simulink model "Octocopter2DLin"  (R2017b)
settings: Solver=VariableStepAuto  StartTime=0.0  StopTime=20  RelTol=1e-3
undefined symbols (not defined in the file): A, ACmp, B1, B2, BCmp, C2, CCmp, D21, DCmp, xInit
settings Model: Creator=jeremie  LastModifiedBy=jeremie

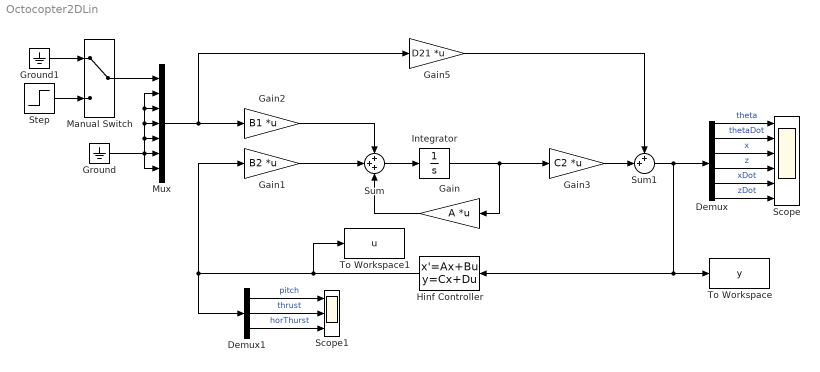
== system Octocopter2DLin ==
  Demux : Demux  Outputs=6
  Demux1 : Demux  Outputs=3
  Gain : Gain  Gain=A  Multiplication=Matrix(K*u)
  Gain1 : Gain  Gain=B2  Multiplication=Matrix(K*u)
  Gain2 : Gain  Gain=B1  Multiplication=Matrix(K*u)
  Gain3 : Gain  Gain=C2  Multiplication=Matrix(K*u)
  Gain5 : Gain  Gain=D21  Multiplication=Matrix(K*u)
  Ground : Ground
  Ground1 : Ground
  Hinf Controller : StateSpace  A=ACmp  B=BCmp  C=CCmp  D=DCmp  InitialCondition=0
  Integrator : Integrator  InitialCondition=xInit
  Manual Switch : ManualSwitch
  Mux : Mux  Inputs=7
  Scope : Scope  NumInputPorts=6
  Scope1 : Scope  NumInputPorts=3
  Step : Step  Time=10  SampleTime=0
  Sum : Sum  Inputs=+++
  Sum1 : Sum  Inputs=++|
  To Workspace : ToWorkspace  VariableName=y  SampleTime=-1
  To Workspace1 : ToWorkspace  VariableName=u  SampleTime=-1
  wires:
  Gain/1 -> Sum/3
  Integrator/1 -> Gain/1, Gain3/1
  Gain1/1 -> Sum/2
  Gain2/1 -> Sum/1
  Sum/1 -> Integrator/1
  Gain3/1 -> Sum1/2
  Gain5/1 -> Sum1/1
  Sum1/1 -> Hinf Controller/1, To Workspace/1, Demux/1
  Hinf Controller/1 -> To Workspace1/1, Gain1/1, Demux1/1
  Mux/1 -> Gain2/1, Gain5/1
  Ground/1 -> Mux/2, Mux/3, Mux/4, Mux/5, Mux/7, Mux/6
  Demux/1 -> Scope/1  "theta"
  Demux/2 -> Scope/2  "thetaDot"
  Demux/3 -> Scope/3  "x"
  Demux/4 -> Scope/4  "z"
  Demux/5 -> Scope/5  "xDot"
  Demux/6 -> Scope/6  "zDot"
  Step/1 -> Manual Switch/2
  Demux1/1 -> Scope1/1  "pitch"
  Demux1/2 -> Scope1/2  "thrust"
  Demux1/3 -> Scope1/3  "horThurst"
  Manual Switch/1 -> Mux/1
  Ground1/1 -> Manual Switch/1
